simulink model "same_probability_model"  (R2024b)
settings: Solver=VariableStepAuto  StartTime=0.0  StopTime=Tsim  RelTol=1e-3
undefined symbols (not defined in the file): Control_pA, Kc, Kg, m, n, p_a, seed
settings Model: Creator=rgivo  LastModifiedBy=rgivo
settings DataIOCC: ReturnWorkspaceOutputs=off

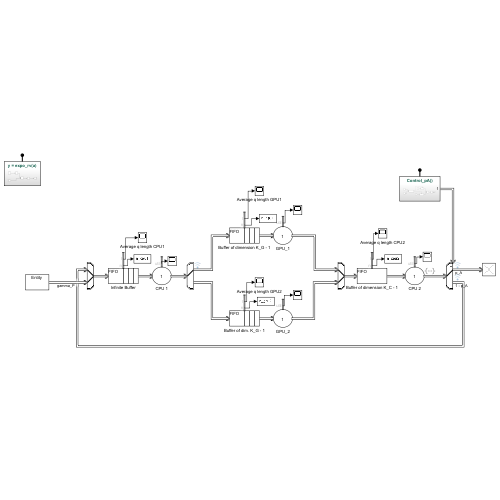
[thumbnail: Simulink's stored preview of the top-level diagram]
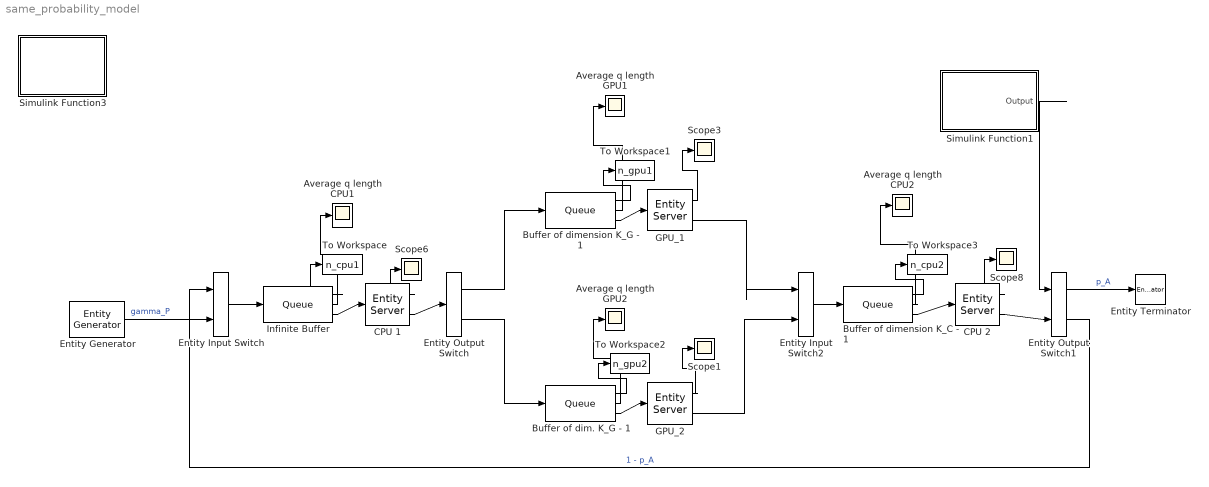
== system same_probability_model ==
  Average q length CPU1 : Scope
  Average q length CPU2 : Scope
  Average q length GPU1 : Scope
  Average q length GPU2 : Scope
  Buffer of dim. K_G - 1 : Queue  InputPortMessageModes=m  OutputPortMessageModes=n,n,m  Capacity=Kg - 1  NumberEntitiesInBlock=on  AverageQueueLength=on
      settings: OutputPortMap=o1,o3,o5
  Buffer of dimension K_C - 1 : Queue  InputPortMessageModes=m  OutputPortMessageModes=n,n,m  Capacity=Kc - 1  NumberEntitiesInBlock=on  AverageQueueLength=on
      settings: OutputPortMap=o1,o3,o5
  Buffer of dimension K_G - 1 : Queue  InputPortMessageModes=m  OutputPortMessageModes=n,n,m  Capacity=Kg-1  NumberEntitiesInBlock=on  AverageQueueLength=on
      settings: OutputPortMap=o1,o3,o5
  CPU 1 : EntityServer  InputPortMessageModes=m  OutputPortMessageModes=n,m  Capacity=1  ServiceTimeSource=MATLAB action  ServiceTimeAction=dt = expo_rv(mu_c);  Utilization=on
      settings: OutputPortMap=o5,o9
  CPU 2 : EntityServer  InputPortMessageModes=m  OutputPortMessageModes=n,m  Capacity=1  ServiceTimeSource=MATLAB action  ServiceTimeAction=dt = expo_rv(mu_c);  ExitAction=Control_pA();  Utilization=on
      settings: OutputPortMap=o5,o9
  Entity Input Switch : EntityInputSwitch  InputPortMessageModes=m,m  OutputPortMessageModes=m
  Entity Input Switch2 : EntityInputSwitch  InputPortMessageModes=m,m  OutputPortMessageModes=m
  Entity Output Switch : EntityOutputSwitch  InputPortMessageModes=m  OutputPortMessageModes=m,m  SwitchingCriterion=Equiprobable  Seed=seed  SwitchAttributeName=Attribute1  InitialPortSelection=2
  Entity Output Switch1 : EntityOutputSwitch  InputPortMessageModes=m,m  OutputPortMessageModes=m,m  SwitchingCriterion=From control port  SwitchAttributeName=Attribute1
      settings: InputPortMap=u0,u1
  Entity Generator : EntityGenerator  OutputPortMessageModes=m  TimeSource=MATLAB action  IntergenerationTimeAction=dt = expo_rv(gamma_p);  GenerateEntityAtSimulationStart=off  EntityType=Structured  EntityTypeName=Entity
  Entity Terminator : EntityTerminator  InputPortMessageModes=m
  GPU_1 : EntityServer  InputPortMessageModes=m  OutputPortMessageModes=n,m  Capacity=1  ServiceTimeSource=MATLAB action  ServiceTimeAction=dt = expo_rv(mu_g);  Utilization=on
      settings: OutputPortMap=o5,o9
  GPU_2 : EntityServer  InputPortMessageModes=m  OutputPortMessageModes=n,m  Capacity=1  ServiceTimeSource=MATLAB action  ServiceTimeAction=dt = expo_rv(mu_g);  Utilization=on
      settings: OutputPortMap=o5,o9
  Infinite Buffer : Queue  InputPortMessageModes=m  OutputPortMessageModes=n,n,m  Capacity=inf  NumberEntitiesInBlock=on  AverageQueueLength=on
      settings: OutputPortMap=o1,o3,o5
  Scope{1,3,6,8} (4 alike) : Scope
  Simulink Function1 : Subsystem  TreatAsAtomicUnit=on
  Simulink Function3 : Subsystem  TreatAsAtomicUnit=on
  To Workspace : ToWorkspace  VariableName=n_cpu1  SaveFormat=Timeseries  SampleTime=-1
  To Workspace1 : ToWorkspace  VariableName=n_gpu1  SaveFormat=Timeseries  SampleTime=-1
  To Workspace2 : ToWorkspace  VariableName=n_gpu2  SaveFormat=Timeseries  SampleTime=-1
  To Workspace3 : ToWorkspace  VariableName=n_cpu2  SaveFormat=Timeseries  SampleTime=-1
  wires:
  Simulink Function1/1(Output) -> Entity Output Switch1/1
  Entity Generator/1 -> Entity Input Switch/2  "gamma_P"
  Buffer of dim. K_G - 1/2 -> Average q length GPU2/1
  Entity Input Switch/1 -> Infinite Buffer/1
  GPU_2/1 -> Scope1/1
  Buffer of dimension K_G - 1/3 -> GPU_1/1
  CPU 1/2 -> Entity Output Switch/1
  Buffer of dim. K_G - 1/3 -> GPU_2/1
  Infinite Buffer/3 -> CPU 1/1
  GPU_1/1 -> Scope3/1
  CPU 1/1 -> Scope6/1
  Buffer of dimension K_G - 1/2 -> Average q length GPU1/1
  Entity Output Switch/2 -> Buffer of dim. K_G - 1/1
  Entity Output Switch/1 -> Buffer of dimension K_G - 1/1
  GPU_1/2 -> Entity Input Switch2/1
  GPU_2/2 -> Entity Input Switch2/2
  CPU 2/1 -> Scope8/1
  Buffer of dimension K_C - 1/3 -> CPU 2/1
  Entity Input Switch2/1 -> Buffer of dimension K_C - 1/1
  CPU 2/2 -> Entity Output Switch1/2
  Entity Output Switch1/1 -> Entity Terminator/1  "p_A"
  Entity Output Switch1/2 -> Entity Input Switch/1  "1 - p_A"
  Infinite Buffer/2 -> Average q length CPU1/1
  Infinite Buffer/1 -> To Workspace/1
  Buffer of dimension K_C - 1/2 -> Average q length CPU2/1
  Buffer of dimension K_G - 1/1 -> To Workspace1/1
  Buffer of dim. K_G - 1/1 -> To Workspace2/1
  Buffer of dimension K_C - 1/1 -> To Workspace3/1

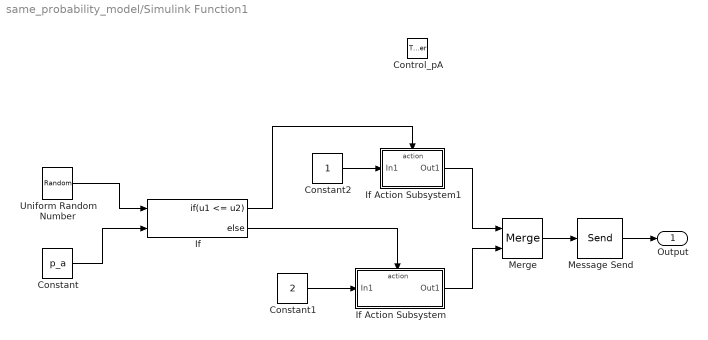
== system same_probability_model/Simulink Function1 ==
  Control_pA : TriggerPort  TriggerType=function-call  IsSimulinkFunction=on  FunctionName=Control_pA  FunctionVisibility=scoped  VariantControl=(inherit)
  Constant : Constant  Value=p_a
  Constant1 : Constant  Value=2
  Constant2 : Constant
  If : If  NumInputs=2  IfExpression=u1 <= u2
  If Action Subsystem : Subsystem  TreatAsAtomicUnit=on
  If Action Subsystem1 : Subsystem  TreatAsAtomicUnit=on
  Merge : Merge
  Message Send : Send  OutputPortMessageModes=m
  Uniform Random Number : UniformRandomNumber  Minimum=0  Seed=seed
  Output : Outport
  wires:
  Uniform Random Number/1 -> If/1
  Constant/1 -> If/2
  If/1 -> If Action Subsystem1/Action
  If/2 -> If Action Subsystem/Action
  Constant2/1 -> If Action Subsystem1/1(In1)
  Constant1/1 -> If Action Subsystem/1(In1)
  If Action Subsystem1/1(Out1) -> Merge/1
  If Action Subsystem/1(Out1) -> Merge/2
  Message Send/1 -> Output/1
  Merge/1 -> Message Send/1

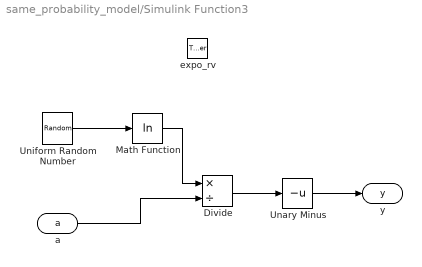
== system same_probability_model/Simulink Function3 ==
  expo_rv : TriggerPort  TriggerType=function-call  IsSimulinkFunction=on  FunctionName=expo_rv  FunctionVisibility=scoped  VariantControl=(inherit)
  Divide : Product  Inputs=*/
  Math Function : Math  Operator=log
  Unary Minus : UnaryMinus
  Uniform Random Number : UniformRandomNumber  Minimum=0  Seed=seed
  a : ArgIn  DisableCoverage=on  ArgumentName=a
  y : ArgOut  DisableCoverage=on  ArgumentName=y
  wires:
  Uniform Random Number/1 -> Math Function/1
  Math Function/1 -> Divide/1
  a/1 -> Divide/2
  Divide/1 -> Unary Minus/1
  Unary Minus/1 -> y/1

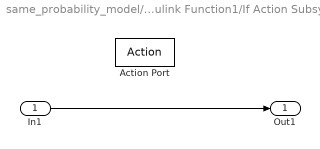
== system same_probability_model/Simulink Function1/If Action Subsystem ==
  In1 : Inport
  Action Port : ActionPort  ActionPortLabel=else
  Out1 : Outport
  wires:
  In1/1 -> Out1/1

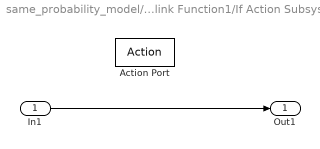
== system same_probability_model/Simulink Function1/If Action Subsystem1 ==
  In1 : Inport
  Action Port : ActionPort  ActionPortLabel=if(u1 <= u2)
  Out1 : Outport
  wires:
  In1/1 -> Out1/1
